simulink model "Arizona_sim_base"  (R2025b)
settings: Solver=VariableStepAuto  StartTime=0.0  StopTime=max(t)  RelTol=1e-3
undefined symbols (not defined in the file): Ts
libraries: cstblocks x6
settings Model: Creator=s158719  LastModifiedBy=thoma
settings SolverCC: AlgebraicLoopSolver=TrustRegion
settings DataIOCC: ReturnWorkspaceOutputs=off
settings DebuggingCC: AlgebraicLoopMsg=none  UnconnectedInputMsg=warning  UnconnectedOutputMsg=warning  UnconnectedLineMsg=warning
settings ModelReferenceCC: EnableRefExpFcnMdlSchedulingChecks=on
settings RTWCC: GPUComputeCapability=3.5  DLArmComputeVersion=19.05

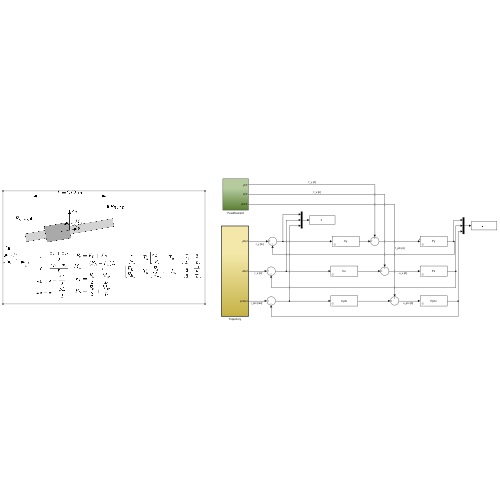
[thumbnail: Simulink's stored preview of the top-level diagram]
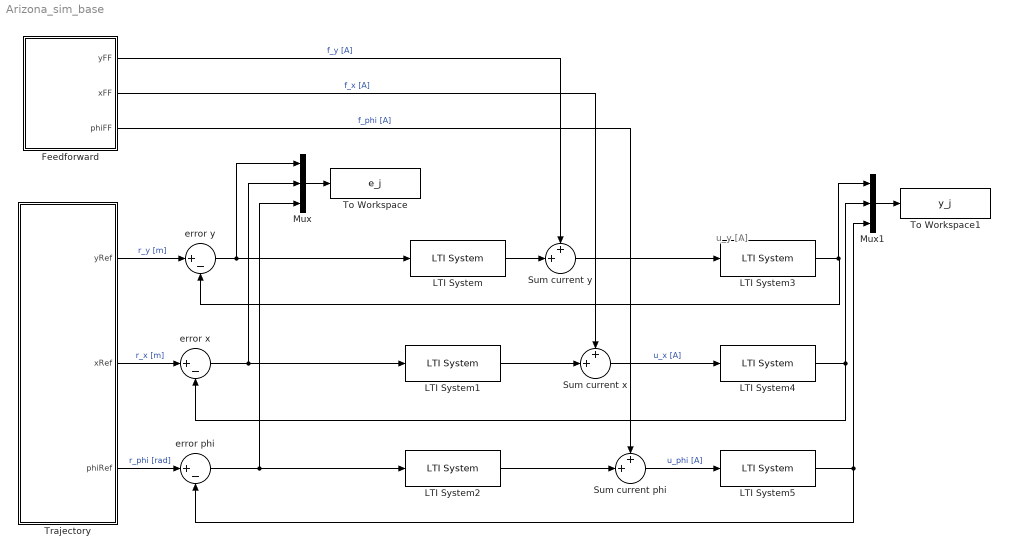
== system Arizona_sim_base ==
  note: u_y [A]
  Feedforward : Subsystem
  LTI System : cstblocks/LTI System  sys=Cy  IC=[]  PadeOrder=0
  LTI System1 : cstblocks/LTI System  sys=Cx  IC=[]  PadeOrder=0
  LTI System2 : cstblocks/LTI System  sys=Cphi  IC=[]  PadeOrder=0
  LTI System3 : cstblocks/LTI System  sys=Py  IC=[]  PadeOrder=0
  LTI System4 : cstblocks/LTI System  sys=Px  IC=[]  PadeOrder=0
  LTI System5 : cstblocks/LTI System  sys=Pphi  IC=[]  PadeOrder=0
  Mux : Mux  Inputs=3
  Mux1 : Mux  Inputs=3
  Sum current phi : Sum  Inputs=++|
  Sum current x : Sum  Inputs=++|
  Sum current y : Sum  Inputs=++|
  To Workspace : ToWorkspace  VariableName=e_j  SampleTime=Ts
      settings: Save2DSignal=2-D array (concatenate along first dimension)
  To Workspace1 : ToWorkspace  VariableName=y_j  SampleTime=Ts
      settings: Save2DSignal=2-D array (concatenate along first dimension)
  Trajectory : Subsystem  TreatAsAtomicUnit=on
  error phi : Sum  Inputs=|+-
  error x : Sum  Inputs=|+-
  error y : Sum  Inputs=|+-
  wires:
  Trajectory/1(yRef) -> error y/1  "r_y [m]"
  Mux1/1 -> To Workspace1/1
  LTI System5/1 -> Mux1/3, error phi/2
  Trajectory/3(phiRef) -> error phi/1  "r_phi [rad]"
  Sum current y/1 -> LTI System3/1
  Sum current x/1 -> LTI System4/1  "u_x [A]"
  Trajectory/2(xRef) -> error x/1  "r_x [m]"
  LTI System3/1 -> Mux1/1, error y/2
  Sum current phi/1 -> LTI System5/1  "u_phi [A]"
  Feedforward/1(yFF) -> Sum current y/1  "f_y [A]"
  Feedforward/3(phiFF) -> Sum current phi/1  "f_phi [A]"
  Feedforward/2(xFF) -> Sum current x/1  "f_x [A]"
  LTI System2/1 -> Sum current phi/2
  Mux/1 -> To Workspace/1
  LTI System1/1 -> Sum current x/2
  LTI System/1 -> Sum current y/2
  LTI System4/1 -> Mux1/2, error x/2
  error y/1 -> LTI System/1, Mux/1
  error x/1 -> LTI System1/1, Mux/2
  error phi/1 -> LTI System2/1, Mux/3

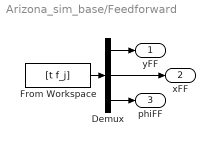
== system Arizona_sim_base/Feedforward ==
  Demux : Demux  Outputs=3
  From Workspace : FromWorkspace  VariableName=[t f_j]  SampleTime=Ts  OutputAfterFinalValue=Setting to zero
  yFF : Outport
  xFF : Outport  Port=2
  phiFF : Outport  Port=3
  wires:
  Demux/3 -> phiFF/1
  From Workspace/1 -> Demux/1
  Demux/1 -> yFF/1
  Demux/2 -> xFF/1

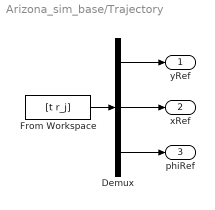
== system Arizona_sim_base/Trajectory ==
  Demux : Demux  Outputs=3
  From Workspace : FromWorkspace  VariableName=[t r_j]  SampleTime=Ts  OutputAfterFinalValue=Holding final value
  yRef : Outport
  xRef : Outport  Port=2
  phiRef : Outport  Port=3
  wires:
  From Workspace/1 -> Demux/1
  Demux/1 -> yRef/1
  Demux/2 -> xRef/1
  Demux/3 -> phiRef/1
